simulink model "FOC_HSMO_G474"  (R2020b)
settings: Solver=FixedStepDiscrete  StartTime=0.0  StopTime=10  FixedStep=TsBSP  RelTol=1e-3
PreLoadFcn:
  | a=1;
values from neighbouring files (symbols this model uses):
  BandwidthCurrentPI = 1256.6370614359173    [G474_FOC_HSMO.sldd]
  GainK = 2.0    [G474_FOC_HSMO.sldd]
  GainM = 0.15    [G474_FOC_HSMO.sldd]
  Ld = 0.000195185    [G474_FOC_HSMO.sldd]    (also in Hall_HSMO_FOC_Data.sldd = 0.0004
  Ld_MODEL = 0.000195185    [G474_FOC_HSMO.sldd]
  Lq = 0.000195185    [G474_FOC_HSMO.sldd]    (also in Hall_HSMO_FOC_Data.sldd = 0.00045
  Lq_MODEL = 0.000195185    [G474_FOC_HSMO.sldd]
  MaxVoltage = 10.0    [G474_FOC_HSMO.sldd]
  PolePairs = 5.0    [G474_FOC_HSMO.sldd]
  PolePairs_MODEL = 5.0    [G474_FOC_HSMO.sldd]
  PWMHalfPeriod = 4199.0    [G474_FOC_HSMO.sldd]
  Rs = 0.1764    [G474_FOC_HSMO.sldd]
  TsBSP = 5.0E-6    [G474_FOC_HSMO.sldd]
  TsFOC = 0.0001    [G474_FOC_HSMO.sldd]
  TsFOC_MODEL = 0.0001    [G474_FOC_HSMO.sldd]
undefined symbols (not defined in the file or in its folder): DiscIntNeverNeededParam, sigbuilder_block
libraries: pid_lib x3, mcbplantlib x1, autolibpmsminterior x1
(part 1 of 2)
PreSaveFcn:
  | cd(fileparts(which(bdroot)));
settings Model: DataDictionary=G474_FOC_HSMO.sldd  PauseTimes=1  PacingRate=1.100000  Creator=beau_  LastModifiedBy=Administrator
settings DataIOCC: SaveOutput=off  DSMLogging=off  SaveTime=off  ReturnWorkspaceOutputs=off
settings OptimizationCC: DefaultParameterBehavior=Inlined  EnhancedBackFolding=on  PassReuseOutputArgsAs=Individual arguments  ZeroExternalMemoryAtStartup=off  OptimizeBlockOrder=speed  DifferentSizesBufferReuse=on  OptimizationCustomize=off  EfficientTunableParamExpr=on
settings DebuggingCC: SignalRangeChecking=warning  ParameterPrecisionLossMsg=none  ParameterTunabilityLossMsg=error
settings HardwareCC: ProdBitPerPointer=32  ProdBitPerSizeT=32  ProdBitPerPtrDiffT=32  ProdLargestAtomicInteger=Long  ProdLargestAtomicFloat=Double  ProdWordSize=32  ProdHWDeviceType=ARM Compatible->ARM Cortex-M
settings SFSimCC: SimParseCustomCode=off  MATLABDynamicMemAlloc=off
settings RTWCC: Description=Embedded Coder  SystemTargetFile=ert.tlc  GenCodeOnly=on  TemplateMakefile=ert_default_tmf  RTWUseSimCustomCode=on
settings CodeAppCC: ForceParamTrailComments=on  GenerateComments=off  IgnoreCustomStorageClasses=off  OperatorAnnotations=on  SimulinkDataObjDesc=on  SFDataObjDesc=on  InsertBlockDesc=on
settings ERTTargetCC: TargetLangStandard=C99 (ISO)  CodeReplacementLibrary=ARM Cortex-M  GenerateSampleERTMain=on  SupportAbsoluteTime=off  SupportNonFinite=off  SupportComplex=off  InlinedParameterPlacement=NonHierarchical  ERTCustomFileTemplate=example_file_process.tlc  IndentSize=4

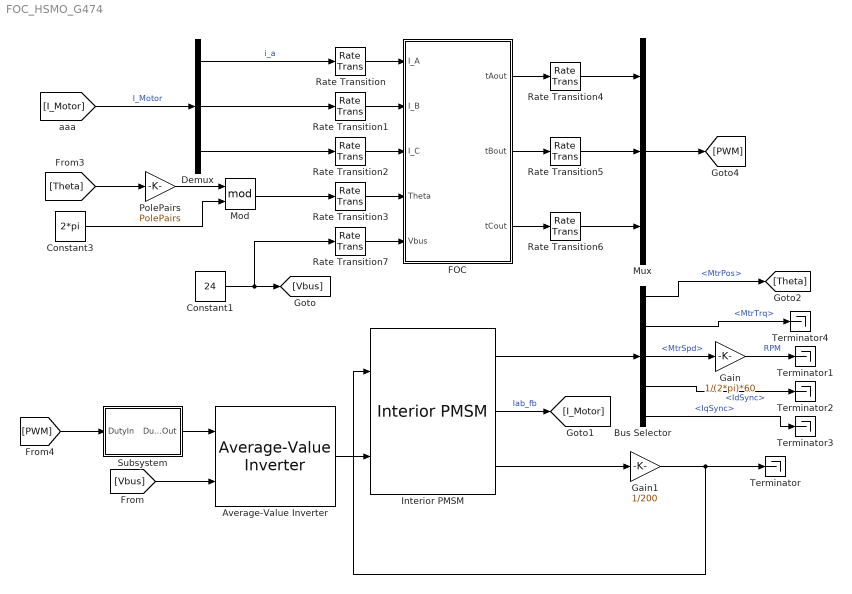
== system FOC_HSMO_G474 ==
  Average-Value Inverter : mcbplantlib/Average-Value Inverter
  Bus Selector : BusSelector  OutputSignals=MtrPos,MtrTrq,MtrSpd,IdSync,IqSync
  Constant1 : Constant  Value=24  SampleTime=TsBSP
  Constant3 : Constant  Value=2*pi  SampleTime=TsBSP
  Demux : Demux  Outputs=3
  FOC : Subsystem  SystemSampleTime=TsFOC
  Gain : Gain  Gain=1/(2*pi)*60
  Gain1 : Gain  Gain=1/200
  Interior PMSM : autolibpmsminterior/Interior PMSM  port_config=Torque  sim_type=Discrete  Ts=TsBSP  P=PolePairs_MODEL  Rs=Rs_MODEL  Ldq=[Ld_MODEL Lq_MODEL]  KConstText=Permanent flux linkage constant (lambda_pm):  lambda_pm=Flux_MODEL  Ke=159.9771  mechanical=[2.8e-4,1e-5,0.01]  idq0=[0 0]  theta_init=0  omega_init=5  KConst=Flux_MODEL  lambda_pm_calc=Flux_MODEL  Kt=0.07  RefBlkName='autolibpmsminterior/Interior PMSM'  aMode=5
      settings: SourceProductBaseCode=PW,MT,UV,VE,VP
  Mod : Math  Operator=mod  SaturateOnIntegerOverflow=on
  Mux : Mux  Inputs=3
  PolePairs : Gain  Gain=PolePairs
  Rate Transition{,1..3,7} (5 alike) : RateTransition
  Rate Transition4 : RateTransition  OutPortSampleTime=TsBSP
  Rate Transition5 : RateTransition  OutPortSampleTime=TsBSP
  Rate Transition6 : RateTransition  OutPortSampleTime=TsBSP
  Subsystem : Subsystem
  Terminator{,1..4} (5 alike) : Terminator
  wires:
  Average-Value Inverter/1 -> Interior PMSM/2
  Rate Transition4/1 -> Mux/1
  Interior PMSM/2 -> [I_Motor]  "Iab_fb"
  Rate Transition7/1 -> FOC/5(Vbus)
  Interior PMSM/3 -> Gain1/1
  Bus Selector/5 -> Terminator3/1  "<IqSync>"
  Bus Selector/4 -> Terminator2/1  "<IdSync>"
  [Vbus] -> Average-Value Inverter/2
  Mux/1 -> [PWM]
  Rate Transition2/1 -> FOC/3(I_C)
  Mod/1 -> Rate Transition3/1
  PolePairs/1 -> Mod/1
  Subsystem/1(DutyOut) -> Average-Value Inverter/1
  Constant1/1 -> Rate Transition7/1, [Vbus]
  Rate Transition3/1 -> FOC/4(Theta)
  Demux/3 -> Rate Transition2/1
  Rate Transition/1 -> FOC/1(I_A)
  Demux/1 -> Rate Transition/1  "i_a"
  Gain1/1 -> Interior PMSM/1, Terminator/1
  Rate Transition5/1 -> Mux/2
  Interior PMSM/1 -> Bus Selector/1
  Rate Transition6/1 -> Mux/3
  Bus Selector/1 -> [Theta]  "<MtrPos>"
  FOC/2(tBout) -> Rate Transition5/1
  [Theta] -> PolePairs/1
  FOC/3(tCout) -> Rate Transition6/1
  FOC/1(tAout) -> Rate Transition4/1
  Demux/2 -> Rate Transition1/1
  Bus Selector/3 -> Gain/1  "<MtrSpd>"
  Constant3/1 -> Mod/2
  Rate Transition1/1 -> FOC/2(I_B)
  [PWM] -> Subsystem/1(DutyIn)
  [I_Motor] -> Demux/1  "I_Motor"
  Gain/1 -> Terminator1/1  "RPM"
  Bus Selector/2 -> Terminator4/1  "<MtrTrq>"

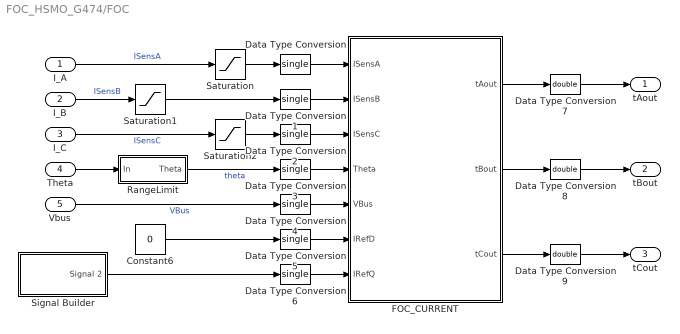
== system FOC_HSMO_G474/FOC ==
  I_A : Inport  OutMin=-100  OutMax=100
  I_B : Inport  Port=2
  I_C : Inport  Port=3
  Theta : Inport  Port=4
  Vbus : Inport  Port=5
  Constant6 : Constant  Value=0  SampleTime=-1
  Data Type Conversion{,1..6} (7 alike) : DataTypeConversion  OutDataTypeStr=single
  Data Type Conversion7 : DataTypeConversion  OutDataTypeStr=double
  Data Type Conversion8 : DataTypeConversion  OutDataTypeStr=double
  Data Type Conversion9 : DataTypeConversion  OutDataTypeStr=double
  FOC_CURRENT : Subsystem  TreatAsAtomicUnit=on  SystemSampleTime=TsFOC_MODEL
  RangeLimit : Subsystem
  Saturation : Saturate  UpperLimit=100  LowerLimit=-100
  Saturation1 : Saturate  UpperLimit=100  LowerLimit=-100
  Saturation2 : Saturate  UpperLimit=100  LowerLimit=-100
  Signal Builder : Subsystem  Tag=STV Subsys  LoadFcn=sigbuilder_block('load');  StartFcn=sigbuilder_block('start');  StopFcn=sigbuilder_block('stop');  ClipboardFcn=sigbuilder_block('clipboard');  mask(Sigbuilder block){tuvar=[0:10]}
      mask help: Simulink:masks:SigbuilderBlock_MD
      mask init:
      | if ~strcmp(get_param(bdroot(gcbh),'SimulationStatus'),'stopped') tuvar = sigbuilder_block('maskInit'); end
      settings: CopyFcn=sigbuilder_block('copy');  DeleteFcn=sigbuilder_block('delete');  ModelCloseFcn=sigbuilder_block('modelClose');  PreSaveFcn=sigbuilder_block('preSave');  PauseFcn=sigbuilder_block('pause');  ContinueFcn=sigbuilder_block('continue');  NameChangeFcn=sigbuilder_block('namechange');  OpenFcn=sigbuilder_block('open',[163.5 909 1141.5 540 ]);  CloseFcn=sigbuilder_block('close');
      mask Display: plot(0, 0, 100, 100,[2, 2, 32, 32, 2], [68, 8, 8, 68, 68],[32, 2], [38, 38], [32, 19, 2],[53, 60, 44], [32, 17, 17, 2],[16, 16, 31, 31]);txt = getActiveGroup(gcbh);text(2, 100, txt,'verticalAlignment', 'top');
  tAout : Outport
  tBout : Outport  Port=2
  tCout : Outport  Port=3
  wires:
  I_A/1 -> Saturation/1  "ISensA"
  I_C/1 -> Saturation2/1  "ISensC"
  Vbus/1 -> Data Type Conversion4/1  "VBus"
  I_B/1 -> Saturation1/1  "ISensB"
  Constant6/1 -> Data Type Conversion5/1
  Theta/1 -> RangeLimit/1(In)
  FOC_CURRENT/3(tCout) -> Data Type Conversion9/1
  FOC_CURRENT/1(tAout) -> Data Type Conversion7/1
  FOC_CURRENT/2(tBout) -> Data Type Conversion8/1
  Saturation/1 -> Data Type Conversion/1
  Saturation1/1 -> Data Type Conversion1/1
  Saturation2/1 -> Data Type Conversion2/1
  RangeLimit/1(Theta) -> Data Type Conversion3/1  "theta"
  Signal Builder/1(Signal 2) -> Data Type Conversion6/1
  Data Type Conversion/1 -> FOC_CURRENT/1(ISensA)
  Data Type Conversion1/1 -> FOC_CURRENT/2(ISensB)
  Data Type Conversion2/1 -> FOC_CURRENT/3(ISensC)
  Data Type Conversion3/1 -> FOC_CURRENT/4(Theta)
  Data Type Conversion4/1 -> FOC_CURRENT/5(VBus)
  Data Type Conversion5/1 -> FOC_CURRENT/6(IRefD)
  Data Type Conversion6/1 -> FOC_CURRENT/7(IRefQ)
  Data Type Conversion7/1 -> tAout/1
  Data Type Conversion8/1 -> tBout/1
  Data Type Conversion9/1 -> tCout/1

== system FOC_HSMO_G474/Subsystem ==
  DutyIn : Inport
  Constant : Constant  Value=0.5  SampleTime=TsBSP
  Gain : Gain  Gain=1/PWMHalfPeriod  ParamDataTypeStr=single
  Gain1 : Gain  Gain=-1
  Sum : Sum  Inputs=|+-
  Sum1 : Sum  Inputs=|++
  DutyOut : Outport
  wires:
  Sum/1 -> Gain1/1
  Constant/1 -> Sum1/2, Sum/2
  DutyIn/1 -> Gain/1
  Gain1/1 -> Sum1/1
  Sum1/1 -> DutyOut/1
  Gain/1 -> Sum/1

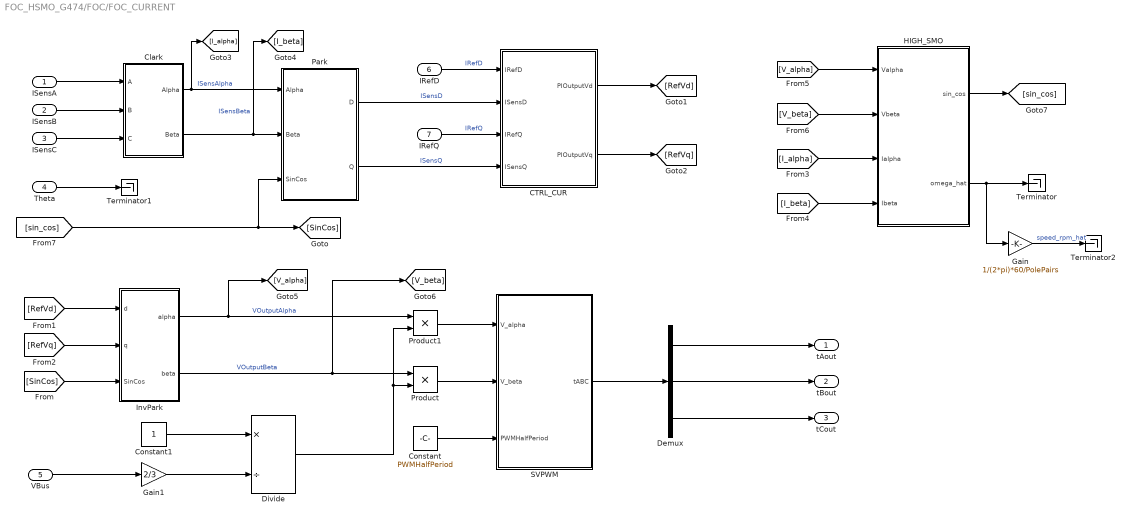
== system FOC_HSMO_G474/FOC/FOC_CURRENT ==
  ISensA : Inport  OutMin=-100  OutMax=100
  ISensB : Inport  Port=2  OutMin=-100  OutMax=100
  ISensC : Inport  Port=3  OutMin=-100  OutMax=100
  Theta : Inport  Port=4  OutMin=-2*pi  OutMax=2*pi
  VBus : Inport  Port=5  OutMin=0  OutMax=500
  IRefD : Inport  Port=6  OutMin=-50  OutMax=50
  IRefQ : Inport  Port=7  OutMin=-50  OutMax=50
  CTRL_CUR : Subsystem  TreatAsAtomicUnit=on
  Clark : Subsystem  TreatAsAtomicUnit=on
      settings: RTWSystemCode=Inline  RTWFcnNameOpts=Use subsystem name
      mask Display:
      | port_label('input',1,'a','texmode','on');
      | port_label('input',2,'b','texmode','on');
      | port_label('input',3,'c','texmode','on');
      | 
      | port_label('output',1,'\alpha','texmode','on');
      | port_label('output',2,'\beta','texmode','on');
      | 
      | fprintf('Clark');
  Constant : Constant  Value=PWMHalfPeriod  OutDataTypeStr=single  SampleTime=-1
  Constant1 : Constant  OutDataTypeStr=single  SampleTime=-1
  Demux : Demux  Outputs=3
  Divide : Product  Inputs=*/
  Gain : Gain  Gain=1/(2*pi)*60/PolePairs
  Gain1 : Gain  Gain=2/3
  HIGH_SMO : Subsystem
      mask Display:
      | port_label('input',1,'U_\alpha','texmode','on');
      | port_label('input',2,'U_\beta','texmode','on');
      | port_label('input',3,'I_\alpha','texmode','on');
      | port_label('input',4,'I_\beta','texmode','on');
      | 
      | port_label('output',1,'sin(\theta_e)cos(\theta_e)','texmode','on');
      | port_label('output',2,'\omega_e','texmode','on');
      | 
      | fprintf('HSMO');
  InvPark : Subsystem  TreatAsAtomicUnit=on
      settings: RTWFcnNameOpts=Use subsystem name
      mask Display:
      | port_label('input',1,'d','texmode','on');
      | port_label('input',2,'q','texmode','on');
      | port_label('input',3,'\theta','texmode','on');
      | 
      | port_label('output',1,'\alpha','texmode','on');
      | port_label('output',2,'\beta','texmode','on');
      | 
      | fprintf('Inverse\nPark')
  Park : Subsystem  TreatAsAtomicUnit=on
      settings: RTWFcnNameOpts=Use subsystem name
      mask Display:
      | port_label('input',1,'\alpha','texmode','on');
      | port_label('input',2, '\beta','texmode','on');
      | port_label('input',3, '\theta','texmode','on');
      | 
      | port_label('output',1,'d','texmode','on');
      | port_label('output',2,'q','texmode','on');
      | fprintf('Park');
  Product : Product
  Product1 : Product
  SVPWM : Subsystem  TreatAsAtomicUnit=on
  Terminator : Terminator
  Terminator1 : Terminator
  Terminator2 : Terminator
  tAout : Outport
  tBout : Outport  Port=2
  tCout : Outport  Port=3
  wires:
  Constant1/1 -> Divide/1
  CTRL_CUR/2(PIOutputVq) -> [RefVq]
  [RefVq] -> InvPark/2(q)
  InvPark/1(alpha) -> Product1/1, [V_alpha]  "VOutputAlpha"
  ISensB/1 -> Clark/2(B)
  IRefQ/1 -> CTRL_CUR/3(IRefQ)  "IRefQ"
  Divide/1 -> Product1/2, Product/2
  Product/1 -> SVPWM/2(V_beta)
  Park/2(Q) -> CTRL_CUR/4(ISensQ)  "ISensQ"
  Gain1/1 -> Divide/2
  [SinCos] -> InvPark/3(SinCos)
  IRefD/1 -> CTRL_CUR/1(IRefD)  "IRefD"
  InvPark/2(beta) -> Product/1, [V_beta]  "VOutputBeta"
  [RefVd] -> InvPark/1(d)
  Constant/1 -> SVPWM/3(PWMHalfPeriod)
  Park/1(D) -> CTRL_CUR/2(ISensD)  "ISensD"
  VBus/1 -> Gain1/1
  CTRL_CUR/1(PIOutputVd) -> [RefVd]
  [sin_cos] -> Park/3(SinCos), [SinCos]
  ISensC/1 -> Clark/3(C)
  ISensA/1 -> Clark/1(A)
  Product1/1 -> SVPWM/1(V_alpha)
  SVPWM/1(tABC) -> Demux/1
  Demux/1 -> tAout/1
  Demux/2 -> tBout/1
  Demux/3 -> tCout/1
  Clark/1(Alpha) -> Park/1(Alpha), [I_alpha]  "ISensAlpha"
  Clark/2(Beta) -> [I_beta], Park/2(Beta)  "ISensBeta"
  [I_alpha] -> HIGH_SMO/3(Ialpha)
  [I_beta] -> HIGH_SMO/4(Ibeta)
  [V_alpha] -> HIGH_SMO/1(Valpha)
  [V_beta] -> HIGH_SMO/2(Vbeta)
  HIGH_SMO/1(sin_cos) -> [sin_cos]
  HIGH_SMO/2(omega_hat) -> Gain/1, Terminator/1
  Gain/1 -> Terminator2/1  "speed_rpm_hat"
  Theta/1 -> Terminator1/1

== system FOC_HSMO_G474/FOC/RangeLimit ==
  In : Inport
  Constant : Constant  Value=2*pi  SampleTime=-1
  Constant1 : Constant  Value=0  SampleTime=-1
  If : If  NumInputs=2  IfExpression=u1  ElseIfExpressions=u2
  If Action Subsystem : Subsystem  TreatAsAtomicUnit=on
  If Action Subsystem1 : Subsystem  TreatAsAtomicUnit=on
  If Action Subsystem2 : Subsystem  TreatAsAtomicUnit=on
  Merge : Merge  Inputs=3
  Relational Operator : RelationalOperator  Operator=>  OutDataTypeStr=boolean  RndMeth=Simplest
  Relational Operator1 : RelationalOperator  Operator=<  OutDataTypeStr=boolean  RndMeth=Simplest
  Theta : Outport
  wires:
  Relational Operator/1 -> If/1
  Constant/1 -> Relational Operator/2
  Constant1/1 -> Relational Operator1/2
  In/1 -> Relational Operator1/1, If Action Subsystem2/1(In1), If Action Subsystem1/1(In1), If Action Subsystem/1(In1), Relational Operator/1
  Relational Operator1/1 -> If/2
  Merge/1 -> Theta/1
  If/3 -> If Action Subsystem2/Action
  If/2 -> If Action Subsystem/Action
  If/1 -> If Action Subsystem1/Action
  If Action Subsystem2/1(Out1) -> Merge/1
  If Action Subsystem/1(Out1) -> Merge/2
  If Action Subsystem1/1(Out1) -> Merge/3

== system FOC_HSMO_G474/FOC/Signal Builder ==
  Demux : Demux  Tag=STV Demux  Outputs=1
      settings: DisplayOption=none
  FromWs : FromWorkspace  Tag=STV FromWs  VariableName=tuvar
      SigBuilderData=|
      | common.afterFinalStr = 'Extrapolate'
      | common.sampleTime = 0
      | dataSet.timeRange = [0 10]
      | dataSet.name = 'Group 1'
      | sbobj.Groups.Name = 'Group 1'
      | sbobj.Groups.Signals.Name = 'Signal 2'
      | sbobj.Groups.Signals.XData = [0 0.99 0.99 1.98 1.98 3 3 4 4 5.01 5.01 6 6 7 7.99 7.99 9 9 10]
      | sbobj.Groups.Signals.YData = [2.85 2.85 8.85 8.85 1.55 1.55 2.7 2.7 9.45 5.25 5.3 5.3 0.8 0.8 0.8 9.95 9.95 10 10]
  Signal 2 : Outport  Tag=STV Outport
  wires:
  FromWs/1 -> Demux/1
  Demux/1 -> Signal 2/1

== system FOC_HSMO_G474/FOC/FOC_CURRENT/CTRL_CUR ==
  IRefD : Inport
  ISensD : Inport  Port=2
  IRefQ : Inport  Port=3
  ISensQ : Inport  Port=4
  Constant1 : Constant  Value=Rs*BandwidthCurrentPI  OutDataTypeStr=single  SampleTime=-1
  Constant2 : Constant  Value=Lq*BandwidthCurrentPI  OutDataTypeStr=single  SampleTime=-1
  Constant3 : Constant  Value=Rs*BandwidthCurrentPI  OutDataTypeStr=single  SampleTime=-1
  Constant4 : Constant  Value=Ld*BandwidthCurrentPI  OutDataTypeStr=single  SampleTime=-1
  Discrete PID Controller : pid_lib/PID Controller  Controller=PI  Form=Parallel  TimeDomain=Discrete-time  UseExternalTs=off  SampleTime=-1  IntegratorMethod=Forward Euler  FilterMethod=Forward Euler  ControllerParametersSource=external  P=1  I=1  D=0  UseFilter=off  N=100  TunerSelectOption=Transfer Function Based (PID Tuner App)  ZeroCross=off  InitialConditionSource=internal  InitialConditionForIntegrator=0  InitialConditionForFilter=0  DifferentiatorICPrevScaledInput=0  ExternalReset=none  TrackingMode=off  Kt=1  LimitOutput=on  SatLimitsSource=internal  UpperSaturationLimit=MaxVoltage  LowerSaturationLimit=-MaxVoltage  LinearizeAsGain=off  AntiWindupMode=clamping  Kb=1  POutMin=[]  POutMax=[]  IOutMin=[]  IOutMax=[]  DOutMin=[]  DOutMax=[]  NOutMin=[]  NOutMax=[]  SumOutMin=[]  SumOutMax=[]  SaturationOutDataTypeStr=Inherit: Inherit via back propagation  SaturationOutMin=[]  SaturationOutMax=[]  PParamMin=[]  PParamMax=[]  IParamMin=[]  IParamMax=[]  DParamMin=[]  DParamMax=[]  NParamMin=[]  NParamMax=[]  KbParamMin=[]  KbParamMax=[]  KtParamMin=[]  KtParamMax=[]  KbOutMin=[]  KbOutMax=[]  KtOutMin=[]  KtOutMax=[]  IntegratorOutMin=[]  IntegratorOutMax=[]  FilterOutMin=[]  FilterOutMax=[]  SumI1OutMin=[]  SumI1OutMax=[]  SumI2OutMin=[]  SumI2OutMax=[]  SumI3OutMin=[]  SumI3OutMax=[]  SumI4OutMin=[]  SumI4OutMax=[]  SumDOutMin=[]  SumDOutMax=[]  DifferentiatorOutMin=[]  DifferentiatorOutMax=[]  FilterDiffOutCoefMin=[]  FilterDiffOutCoefMax=[]  ReciprocalOutMin=[]  ReciprocalOutMax=[]  SumDenOutMin=[]  SumDenOutMax=[]  SumNumOutMin=[]  SumNumOutMax=[]  DivideOutMin=[]  DivideOutMax=[]  UdiffTsProdOutMin=[]  UdiffTsProdOutMax=[]  NTsProdOutMin=[]  NTsProdOutMax=[]  UintegralTsProdOutMin=[]  UintegralTsProdOutMax=[]  UngainTsProdOutMin=[]  UngainTsProdOutMax=[]  IntegratorContinuousStateAttributes=''  IntegratorStateMustResolveToSignalObject=off  IntegratorRTWStateStorageClass=Auto  FilterContinuousStateAttributes=''  FilterStateMustResolveToSignalObject=off  FilterRTWStateStorageClass=Auto  ParallelPVariant=ExternalParameters  IdealPVariant=Disabled  IVariant=ExternalParameters  DVariant=Disabled  IntegratorVariant=Discrete  SatVariant=Enabled  AWVariant=DiscClampingParallel  PCopyVariant=Disabled  TRVariant=Disabled  FdbkBlocksVariant=Forward  IdealPFdbkVariant=Disabled  SatFdbkVariant=Disabled  DerivativeFilterVariant=Disabled  NVariant=Disabled  NCopyVariant=Disabled_SignalSpec  FilterICVariant=Disabled  IntegratorICVariant=InternalICs  ExternalResetVariant=Disabled  TRSumVariant=Passthrough  SumFdbkVariant=Disabled  SumVariant=Sum_PI  TsampFilterVariant=InternalTs  TsampNgainVariant=Passthrough  TsampIntegralVariant=Passthrough  ExternalSaturationOutDataTypeStr=Inherit: Same as second input
  Discrete PID Controller1 : pid_lib/PID Controller  Controller=PI  Form=Parallel  TimeDomain=Discrete-time  UseExternalTs=off  SampleTime=-1  IntegratorMethod=Forward Euler  FilterMethod=Forward Euler  ControllerParametersSource=external  P=1  I=1  D=0  UseFilter=off  N=100  TunerSelectOption=Transfer Function Based (PID Tuner App)  ZeroCross=off  InitialConditionSource=internal  InitialConditionForIntegrator=0  InitialConditionForFilter=0  DifferentiatorICPrevScaledInput=0  ExternalReset=none  TrackingMode=off  Kt=1  LimitOutput=on  SatLimitsSource=internal  UpperSaturationLimit=MaxVoltage  LowerSaturationLimit=-MaxVoltage  LinearizeAsGain=off  AntiWindupMode=clamping  Kb=1  POutMin=[]  POutMax=[]  IOutMin=[]  IOutMax=[]  DOutMin=[]  DOutMax=[]  NOutMin=[]  NOutMax=[]  SumOutMin=[]  SumOutMax=[]  SaturationOutDataTypeStr=Inherit: Inherit via back propagation  SaturationOutMin=[]  SaturationOutMax=[]  PParamMin=[]  PParamMax=[]  IParamMin=[]  IParamMax=[]  DParamMin=[]  DParamMax=[]  NParamMin=[]  NParamMax=[]  KbParamMin=[]  KbParamMax=[]  KtParamMin=[]  KtParamMax=[]  KbOutMin=[]  KbOutMax=[]  KtOutMin=[]  KtOutMax=[]  IntegratorOutMin=[]  IntegratorOutMax=[]  FilterOutMin=[]  FilterOutMax=[]  SumI1OutMin=[]  SumI1OutMax=[]  SumI2OutMin=[]  SumI2OutMax=[]  SumI3OutMin=[]  SumI3OutMax=[]  SumI4OutMin=[]  SumI4OutMax=[]  SumDOutMin=[]  SumDOutMax=[]  DifferentiatorOutMin=[]  DifferentiatorOutMax=[]  FilterDiffOutCoefMin=[]  FilterDiffOutCoefMax=[]  ReciprocalOutMin=[]  ReciprocalOutMax=[]  SumDenOutMin=[]  SumDenOutMax=[]  SumNumOutMin=[]  SumNumOutMax=[]  DivideOutMin=[]  DivideOutMax=[]  UdiffTsProdOutMin=[]  UdiffTsProdOutMax=[]  NTsProdOutMin=[]  NTsProdOutMax=[]  UintegralTsProdOutMin=[]  UintegralTsProdOutMax=[]  UngainTsProdOutMin=[]  UngainTsProdOutMax=[]  IntegratorContinuousStateAttributes=''  IntegratorStateMustResolveToSignalObject=off  IntegratorRTWStateStorageClass=Auto  FilterContinuousStateAttributes=''  FilterStateMustResolveToSignalObject=off  FilterRTWStateStorageClass=Auto  ParallelPVariant=ExternalParameters  IdealPVariant=Disabled  IVariant=ExternalParameters  DVariant=Disabled  IntegratorVariant=Discrete  SatVariant=Enabled  AWVariant=DiscClampingParallel  PCopyVariant=Disabled  TRVariant=Disabled  FdbkBlocksVariant=Forward  IdealPFdbkVariant=Disabled  SatFdbkVariant=Disabled  DerivativeFilterVariant=Disabled  NVariant=Disabled  NCopyVariant=Disabled_SignalSpec  FilterICVariant=Disabled  IntegratorICVariant=InternalICs  ExternalResetVariant=Disabled  TRSumVariant=Passthrough  SumFdbkVariant=Disabled  SumVariant=Sum_PI  TsampFilterVariant=InternalTs  TsampNgainVariant=Passthrough  TsampIntegralVariant=Passthrough  ExternalSaturationOutDataTypeStr=Inherit: Same as second input
  Sum : Sum  Inputs=|+-
  Sum1 : Sum  Inputs=|+-
  PIOutputVd : Outport
  PIOutputVq : Outport  Port=2
  wires:
  IRefD/1 -> Sum/1
  Sum/1 -> Discrete PID Controller/1
  Discrete PID Controller/1 -> PIOutputVd/1  "PIOutputVd"
  ISensD/1 -> Sum/2
  Constant4/1 -> Discrete PID Controller/2
  Constant3/1 -> Discrete PID Controller/3
  IRefQ/1 -> Sum1/1
  Constant2/1 -> Discrete PID Controller1/2
  Sum1/1 -> Discrete PID Controller1/1
  ISensQ/1 -> Sum1/2
  Constant1/1 -> Discrete PID Controller1/3
  Discrete PID Controller1/1 -> PIOutputVq/1  "PIOutputVq"

== system FOC_HSMO_G474/FOC/FOC_CURRENT/Clark ==
  A : Inport
  B : Inport  Port=2
  C : Inport  Port=3
  Gain : Gain  Gain=single(2/3)
  Gain1 : Gain  Gain=0.5
  Gain2 : Gain  Gain=single(sqrt(3)/3)
  Sum : Sum  Inputs=|++
  Sum1 : Sum  Inputs=|+-
  Sum2 : Sum  Inputs=+-|
  Alpha : Outport
  Beta : Outport  Port=2
  wires:
  Sum/1 -> Gain1/1
  Gain2/1 -> Beta/1
  B/1 -> Sum2/1, Sum/1
  Gain1/1 -> Sum1/2
  Gain/1 -> Alpha/1
  Sum2/1 -> Gain2/1
  C/1 -> Sum2/2, Sum/2
  A/1 -> Sum1/1
  Sum1/1 -> Gain/1

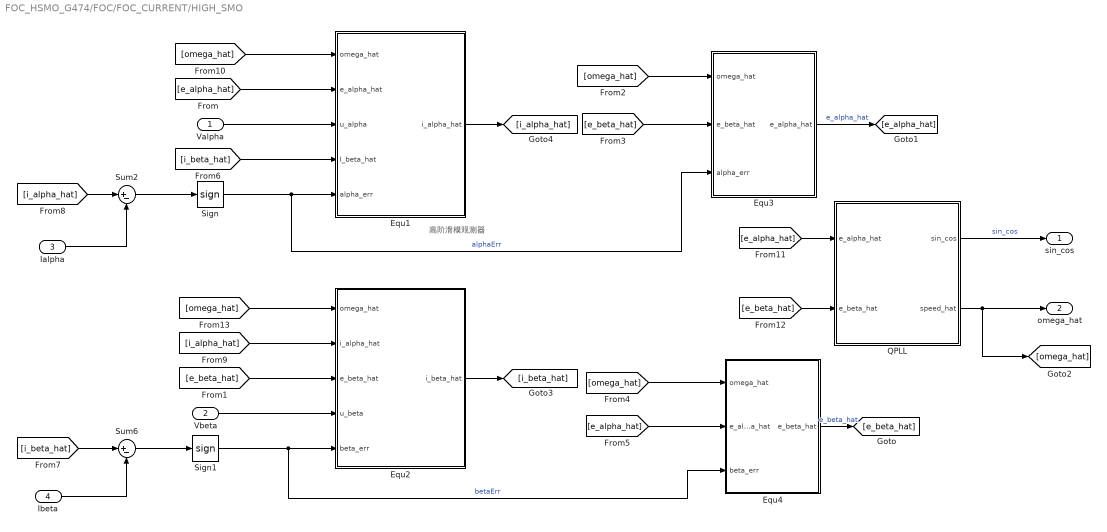
== system FOC_HSMO_G474/FOC/FOC_CURRENT/HIGH_SMO ==
  note: 高阶滑模观测器
  Valpha : Inport
  Vbeta : Inport  Port=2
  Ialpha : Inport  Port=3
  Ibeta : Inport  Port=4
  Equ1 : Subsystem
  Equ2 : Subsystem
  Equ3 : Subsystem
  Equ4 : Subsystem
  QPLL : Subsystem
  Sign : Signum
  Sign1 : Signum
  Sum2 : Sum  Inputs=|+-
  Sum6 : Sum  Inputs=|+-
  sin_cos : Outport
  omega_hat : Outport  Port=2
  wires:
  Sum6/1 -> Sign1/1
  Sum2/1 -> Sign/1
  Sign/1 -> Equ3/3(alpha_err), Equ1/5(alpha_err)  "alphaErr"
  Ialpha/1 -> Sum2/2
  Sign1/1 -> Equ4/3(beta_err), Equ2/5(beta_err)  "betaErr"
  Ibeta/1 -> Sum6/2
  Equ1/1(i_alpha_hat) -> [i_alpha_hat]
  [e_alpha_hat] -> Equ1/2(e_alpha_hat)
  Valpha/1 -> Equ1/3(u_alpha)
  [e_beta_hat] -> Equ2/3(e_beta_hat)
  Vbeta/1 -> Equ2/4(u_beta)
  Equ2/1(i_beta_hat) -> [i_beta_hat]
  [i_beta_hat] -> Equ1/4(I_beta_hat)
  [i_beta_hat] -> Sum6/1
  [i_alpha_hat] -> Sum2/1
  [i_alpha_hat] -> Equ2/2(i_alpha_hat)
  [omega_hat] -> Equ3/1(omega_hat)
  [e_beta_hat] -> Equ3/2(e_beta_hat)
  [omega_hat] -> Equ4/1(omega_hat)
  [e_alpha_hat] -> Equ4/2(e_alpha_hat)
  [omega_hat] -> Equ1/1(omega_hat)
  Equ4/1(e_beta_hat) -> [e_beta_hat]  "e_beta_hat"
  Equ3/1(e_alpha_hat) -> [e_alpha_hat]  "e_alpha_hat"
  [e_alpha_hat] -> QPLL/1(e_alpha_hat)
  [e_beta_hat] -> QPLL/2(e_beta_hat)
  QPLL/2(speed_hat) -> [omega_hat], omega_hat/1
  QPLL/1(sin_cos) -> sin_cos/1  "sin_cos"
  [omega_hat] -> Equ2/1(omega_hat)

== system FOC_HSMO_G474/FOC/FOC_CURRENT/InvPark ==
  d : Inport
  q : Inport  Port=2
  SinCos : Inport  Port=3
  Demux : Demux  Outputs=2
  Product{,1..3} (4 alike) : Product
  Sum : Sum  Inputs=|+-
  Sum1 : Sum  Inputs=|++
  alpha : Outport
  beta : Outport  Port=2
  wires:
  Sum/1 -> alpha/1
  SinCos/1 -> Demux/1
  d/1 -> Product2/1, Product/1
  Demux/2 -> Product/2, Product3/2
  q/1 -> Product3/1, Product1/1
  Demux/1 -> Product1/2, Product2/2
  Product/1 -> Sum/1
  Product1/1 -> Sum/2
  Product2/1 -> Sum1/1
  Product3/1 -> Sum1/2
  Sum1/1 -> beta/1

== system FOC_HSMO_G474/FOC/FOC_CURRENT/Park ==
  Alpha : Inport
  Beta : Inport  Port=2
  SinCos : Inport  Port=3
  Demux : Demux  Outputs=2
  Product{,1..3} (4 alike) : Product
  Sum : Sum  Inputs=|++
  Sum1 : Sum  Inputs=|-+
  D : Outport
  Q : Outport  Port=2
  wires:
  Beta/1 -> Product3/1, Product1/1
  Alpha/1 -> Product2/1, Product/1
  SinCos/1 -> Demux/1
  Demux/2 -> Product/2, Product3/2
  Demux/1 -> Product1/2, Product2/2
  Product/1 -> Sum/1
  Product1/1 -> Sum/2
  Sum/1 -> D/1
  Product2/1 -> Sum1/1
  Product3/1 -> Sum1/2
  Sum1/1 -> Q/1

== system FOC_HSMO_G474/FOC/FOC_CURRENT/SVPWM ==
  V_alpha : Inport
  V_beta : Inport  Port=2
  PWMHalfPeriod : Inport  Port=3
  CalcPWM : Subsystem
  JudgeSector : Subsystem
  tABC : Outport
  wires:
  V_alpha/1 -> CalcPWM/1(u_alpha_prime), JudgeSector/1(u_alpha_prime)
  V_beta/1 -> CalcPWM/2(u_beta_prime), JudgeSector/2(u_beta_prime)
  JudgeSector/1(sector) -> CalcPWM/3(sector)
  CalcPWM/1(tABC) -> tABC/1
  PWMHalfPeriod/1 -> CalcPWM/4(Tpwm)

== system FOC_HSMO_G474/FOC/RangeLimit/If Action Subsystem ==
  In1 : Inport
  Action Port : ActionPort  ActionPortLabel=elseif(u2)
  Constant : Constant  Value=2*pi  SampleTime=-1
  Sum : Sum  Inputs=|++
  Out1 : Outport
  wires:
  In1/1 -> Sum/1
  Constant/1 -> Sum/2
  Sum/1 -> Out1/1

== system FOC_HSMO_G474/FOC/RangeLimit/If Action Subsystem1 ==
  In1 : Inport
  Action Port : ActionPort  ActionPortLabel=if(u1)
  Constant : Constant  Value=2*pi  SampleTime=-1
  Sum : Sum  Inputs=|+-
  Out1 : Outport
  wires:
  In1/1 -> Sum/1
  Constant/1 -> Sum/2
  Sum/1 -> Out1/1

== system FOC_HSMO_G474/FOC/RangeLimit/If Action Subsystem2 ==
  In1 : Inport
  Action Port : ActionPort  ActionPortLabel=else
  Out1 : Outport
  wires:
  In1/1 -> Out1/1

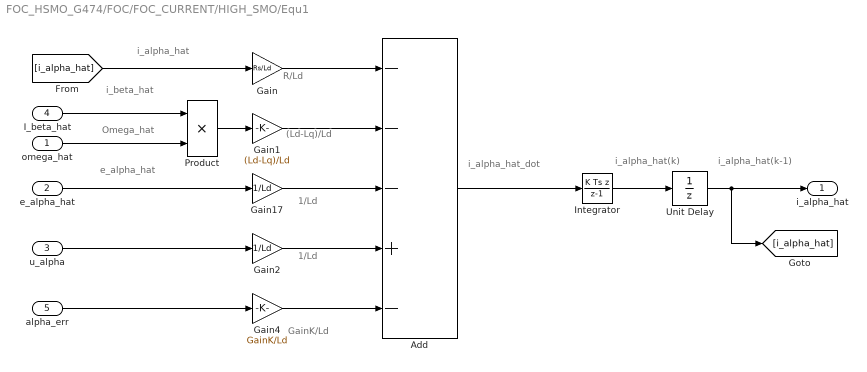
== system FOC_HSMO_G474/FOC/FOC_CURRENT/HIGH_SMO/Equ1 ==
  note: i_alpha_hat(k)
  note: GainK/Ld
  note: i_alpha_hat
  note: R/Ld
  note: (Ld-Lq)/Ld
  note: i_alpha_hat_dot
  note: 1/Ld
  note: e_alpha_hat
  note: 1/Ld
  note: i_beta_hat
  note: Omega_hat
  note: i_alpha_hat(k-1)
  omega_hat : Inport
  e_alpha_hat : Inport  Port=2
  u_alpha : Inport  Port=3
  I_beta_hat : Inport  Port=4
  alpha_err : Inport  Port=5
  Add : Sum  Inputs=---+-
  Gain : Gain  Gain=Rs/Ld
  Gain1 : Gain  Gain=(Ld-Lq)/Ld
  Gain17 : Gain  Gain=1/Ld
  Gain2 : Gain  Gain=1/Ld
  Gain4 : Gain  Gain=GainK/Ld
  Integrator : DiscreteIntegrator  IntegratorMethod=Integration: Backward Euler  SampleTime=-1  ICPrevOutput=DiscIntNeverNeededParam  ICPrevScaledInput=DiscIntNeverNeededParam  mask(DiscretizedDiscreteIntegrator){}
      mask init:
      | %tustin
  Product : Product
  Unit Delay : UnitDelay  SampleTime=-1  HasFrameUpgradeWarning=on
  i_alpha_hat : Outport
  wires:
  Gain1/1 -> Add/2
  Gain4/1 -> Add/5
  Product/1 -> Gain1/1
  Add/1 -> Integrator/1
  I_beta_hat/1 -> Product/1
  Unit Delay/1 -> [i_alpha_hat], i_alpha_hat/1
  Gain/1 -> Add/1
  u_alpha/1 -> Gain2/1
  Gain2/1 -> Add/4
  Integrator/1 -> Unit Delay/1
  omega_hat/1 -> Product/2
  Gain17/1 -> Add/3
  e_alpha_hat/1 -> Gain17/1
  alpha_err/1 -> Gain4/1
  [i_alpha_hat] -> Gain/1

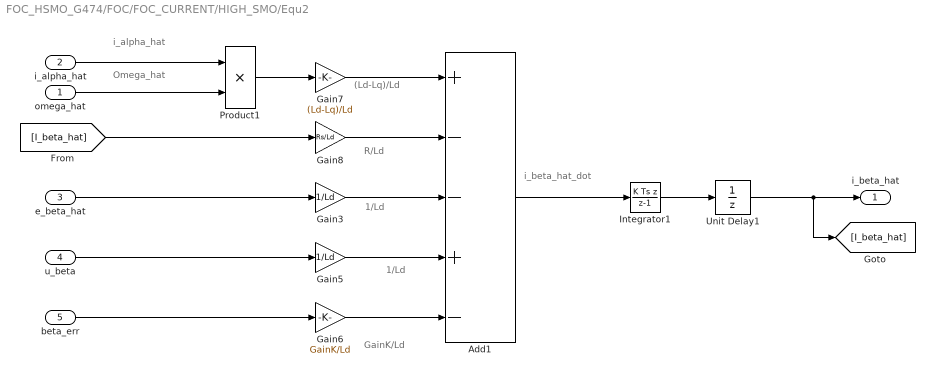
== system FOC_HSMO_G474/FOC/FOC_CURRENT/HIGH_SMO/Equ2 ==
  note: R/Ld
  note: (Ld-Lq)/Ld
  note: 1/Ld
  note: i_alpha_hat
  note: Omega_hat
  note: 1/Ld
  note: GainK/Ld
  note: i_beta_hat_dot
  omega_hat : Inport
  i_alpha_hat : Inport  Port=2
  e_beta_hat : Inport  Port=3
  u_beta : Inport  Port=4
  beta_err : Inport  Port=5
  Add1 : Sum  Inputs=+--+-
  Gain3 : Gain  Gain=1/Ld
  Gain5 : Gain  Gain=1/Ld
  Gain6 : Gain  Gain=GainK/Ld
  Gain7 : Gain  Gain=(Ld-Lq)/Ld
  Gain8 : Gain  Gain=Rs/Ld
  Integrator1 : DiscreteIntegrator  IntegratorMethod=Integration: Backward Euler  SampleTime=-1  ICPrevOutput=DiscIntNeverNeededParam  ICPrevScaledInput=DiscIntNeverNeededParam  mask(DiscretizedDiscreteIntegrator){}
      mask init:
      | %tustin
  Product1 : Product
  Unit Delay1 : UnitDelay  SampleTime=-1  HasFrameUpgradeWarning=on
  i_beta_hat : Outport
  wires:
  Gain8/1 -> Add1/2
  u_beta/1 -> Gain5/1
  Add1/1 -> Integrator1/1
  Gain3/1 -> Add1/3
  i_alpha_hat/1 -> Product1/1
  Gain5/1 -> Add1/4
  Gain6/1 -> Add1/5
  Integrator1/1 -> Unit Delay1/1
  Product1/1 -> Gain7/1
  Gain7/1 -> Add1/1
  beta_err/1 -> Gain6/1
  e_beta_hat/1 -> Gain3/1
  Unit Delay1/1 -> [I_beta_hat], i_beta_hat/1
  omega_hat/1 -> Product1/2
  [I_beta_hat] -> Gain8/1

== system FOC_HSMO_G474/FOC/FOC_CURRENT/HIGH_SMO/Equ3 ==
  note: GainM/Ld
  note: e_alpha_hat_dot
  omega_hat : Inport
  e_beta_hat : Inport  Port=2
  alpha_err : Inport  Port=3
  Add2 : Sum  Inputs=-+
  Gain9 : Gain  Gain=GainM/Ld
  Integrator2 : DiscreteIntegrator  IntegratorMethod=Integration: Backward Euler  SampleTime=-1  ICPrevOutput=DiscIntNeverNeededParam  ICPrevScaledInput=DiscIntNeverNeededParam  mask(DiscretizedDiscreteIntegrator){}
      mask init:
      | %tustin
  Product2 : Product
  Unit Delay2 : UnitDelay  SampleTime=-1  HasFrameUpgradeWarning=on
  e_alpha_hat : Outport
  wires:
  alpha_err/1 -> Gain9/1
  Add2/1 -> Integrator2/1
  Unit Delay2/1 -> e_alpha_hat/1
  omega_hat/1 -> Product2/1
  Product2/1 -> Add2/1
  Integrator2/1 -> Unit Delay2/1
  e_beta_hat/1 -> Product2/2
  Gain9/1 -> Add2/2

== system FOC_HSMO_G474/FOC/FOC_CURRENT/HIGH_SMO/Equ4 ==
  note: GainM/Ld
  note: e_beta_hat_dot
  omega_hat : Inport
  e_alpha_hat : Inport  Port=2
  beta_err : Inport  Port=3
  Add3 : Sum
  Gain10 : Gain  Gain=GainM/Ld
  Integrator3 : DiscreteIntegrator  IntegratorMethod=Integration: Backward Euler  SampleTime=-1  ICPrevOutput=DiscIntNeverNeededParam  ICPrevScaledInput=DiscIntNeverNeededParam  mask(DiscretizedDiscreteIntegrator){}
      mask init:
      | %tustin
  Product3 : Product
  Unit Delay3 : UnitDelay  SampleTime=-1  HasFrameUpgradeWarning=on
  e_beta_hat : Outport
  wires:
  Integrator3/1 -> Unit Delay3/1
  Add3/1 -> Integrator3/1
  Gain10/1 -> Add3/2
  Product3/1 -> Add3/1
  beta_err/1 -> Gain10/1
  Unit Delay3/1 -> e_beta_hat/1
  omega_hat/1 -> Product3/1
  e_alpha_hat/1 -> Product3/2

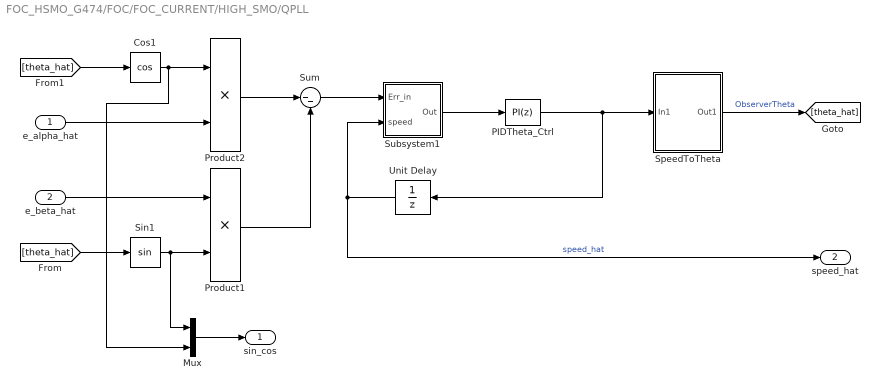
== system FOC_HSMO_G474/FOC/FOC_CURRENT/HIGH_SMO/QPLL ==
  e_alpha_hat : Inport
  e_beta_hat : Inport  Port=2
  Cos1 : Trigonometry  Operator=cos
  Mux : Mux  Inputs=2
  PIDTheta_Ctrl : pid_lib/PID Controller  Controller=PI  Form=Parallel  TimeDomain=Discrete-time  UseExternalTs=off  SampleTime=-1  IntegratorMethod=Forward Euler  FilterMethod=Forward Euler  ControllerParametersSource=internal  P=2*0.707*100  I=100*100  D=0  UseFilter=on  N=100  TunerSelectOption=Transfer Function Based (PID Tuner App)  ZeroCross=off  InitialConditionSource=internal  InitialConditionForIntegrator=1  InitialConditionForFilter=0  DifferentiatorICPrevScaledInput=0  ExternalReset=none  TrackingMode=off  Kt=1  LimitOutput=on  SatLimitsSource=internal  UpperSaturationLimit=2*pi*500  LowerSaturationLimit=-2*pi*500  LinearizeAsGain=off  AntiWindupMode=clamping  Kb=50  POutMin=[]  POutMax=[]  IOutMin=[]  IOutMax=[]  DOutMin=[]  DOutMax=[]  NOutMin=[]  NOutMax=[]  SumOutMin=[]  SumOutMax=[]  SaturationOutDataTypeStr=Inherit: Inherit via back propagation  SaturationOutMin=[]  SaturationOutMax=[]  PParamMin=[]  PParamMax=[]  IParamMin=[]  IParamMax=[]  DParamMin=[]  DParamMax=[]  NParamMin=[]  NParamMax=[]  KbParamMin=[]  KbParamMax=[]  KtParamMin=[]  KtParamMax=[]  KbOutMin=[]  KbOutMax=[]  KtOutMin=[]  KtOutMax=[]  IntegratorOutMin=[]  IntegratorOutMax=[]  FilterOutMin=[]  FilterOutMax=[]  SumI1OutMin=[]  SumI1OutMax=[]  SumI2OutMin=[]  SumI2OutMax=[]  SumI3OutMin=[]  SumI3OutMax=[]  SumI4OutMin=[]  SumI4OutMax=[]  SumDOutMin=[]  SumDOutMax=[]  DifferentiatorOutMin=[]  DifferentiatorOutMax=[]  FilterDiffOutCoefMin=[]  FilterDiffOutCoefMax=[]  ReciprocalOutMin=[]  ReciprocalOutMax=[]  SumDenOutMin=[]  SumDenOutMax=[]  SumNumOutMin=[]  SumNumOutMax=[]  DivideOutMin=[]  DivideOutMax=[]  UdiffTsProdOutMin=[]  UdiffTsProdOutMax=[]  NTsProdOutMin=[]  NTsProdOutMax=[]  UintegralTsProdOutMin=[]  UintegralTsProdOutMax=[]  UngainTsProdOutMin=[]  UngainTsProdOutMax=[]  IntegratorContinuousStateAttributes=''  IntegratorStateMustResolveToSignalObject=off  IntegratorRTWStateStorageClass=Auto  FilterContinuousStateAttributes=''  FilterStateMustResolveToSignalObject=off  FilterRTWStateStorageClass=Auto  ParallelPVariant=InternalParameters  IdealPVariant=Disabled  IVariant=InternalParameters  DVariant=Disabled  IntegratorVariant=Discrete  SatVariant=Enabled  AWVariant=DiscClampingParallel  PCopyVariant=Disabled  TRVariant=Disabled  FdbkBlocksVariant=Forward  IdealPFdbkVariant=Disabled  SatFdbkVariant=Disabled  DerivativeFilterVariant=Disabled  NVariant=Disabled  NCopyVariant=Disabled_SignalSpec  FilterICVariant=Disabled  IntegratorICVariant=InternalICs  ExternalResetVariant=Disabled  TRSumVariant=Passthrough  SumFdbkVariant=Disabled  SumVariant=Sum_PI  TsampFilterVariant=InternalTs  TsampNgainVariant=Passthrough  TsampIntegralVariant=Passthrough  ExternalSaturationOutDataTypeStr=Inherit: Same as second input
  Product1 : Product
  Product2 : Product
  Sin1 : Trigonometry
  SpeedToTheta : Subsystem
  Subsystem1 : Subsystem
  Sum : Sum  Inputs=|--
  Unit Delay : UnitDelay  SampleTime=-1  HasFrameUpgradeWarning=on
  sin_cos : Outport
  speed_hat : Outport  Port=2
  wires:
  Sin1/1 -> Mux/1, Product1/2
  Subsystem1/1(Out) -> PIDTheta_Ctrl/1
  Cos1/1 -> Mux/2, Product2/1
  Sum/1 -> Subsystem1/1(Err_in)
  Product1/1 -> Sum/2
  Product2/1 -> Sum/1
  e_beta_hat/1 -> Product1/1
  e_alpha_hat/1 -> Product2/2
  Unit Delay/1 -> speed_hat/1, Subsystem1/2(speed)  "speed_hat"
  [theta_hat] -> Sin1/1
  [theta_hat] -> Cos1/1
  SpeedToTheta/1(Out1) -> [theta_hat]  "ObserverTheta"
  PIDTheta_Ctrl/1 -> Unit Delay/1, SpeedToTheta/1(In1)
  Mux/1 -> sin_cos/1

== system FOC_HSMO_G474/FOC/FOC_CURRENT/SVPWM/CalcPWM ==
  u_alpha_prime : Inport
  u_beta_prime : Inport  Port=2
  sector : Inport  Port=3
  Tpwm : Inport  Port=4
  Merge : Merge  Inputs=6
  Switch Case : SwitchCase  CaseConditions={1,2,3,4,5,6}  ShowDefaultCase=off
  Switch Case Action Subsystem : Subsystem  TreatAsAtomicUnit=on
  Switch Case Action Subsystem1 : Subsystem  TreatAsAtomicUnit=on
  Switch Case Action Subsystem2 : Subsystem  TreatAsAtomicUnit=on
  Switch Case Action Subsystem3 : Subsystem  TreatAsAtomicUnit=on
  Switch Case Action Subsystem4 : Subsystem  TreatAsAtomicUnit=on
  Switch Case Action Subsystem5 : Subsystem  TreatAsAtomicUnit=on
  tABC : Outport
  wires:
  sector/1 -> Switch Case/1
  Switch Case/1 -> Switch Case Action Subsystem/Action
  u_alpha_prime/1 -> Switch Case Action Subsystem5/1(u_alpha_prime), Switch Case Action Subsystem2/1(u_alpha_prime), Switch Case Action Subsystem1/1(u_alpha_prime), Switch Case Action Subsystem/1(u_alpha_prime), Switch Case Action Subsystem3/1(u_alpha_prime), Switch Case Action Subsystem4/1(u_alpha_prime)
  Tpwm/1 -> Switch Case Action Subsystem5/3(Tpwm), Switch Case Action Subsystem4/3(Tpwm), Switch Case Action Subsystem3/3(Tpwm), Switch Case Action Subsystem2/3(Tpwm), Switch Case Action Subsystem1/3(Tpwm), Switch Case Action Subsystem/3(Tpwm)
  Switch Case/2 -> Switch Case Action Subsystem1/Action
  Switch Case/3 -> Switch Case Action Subsystem2/Action
  Switch Case/4 -> Switch Case Action Subsystem3/Action
  Switch Case/5 -> Switch Case Action Subsystem4/Action
  Switch Case/6 -> Switch Case Action Subsystem5/Action
  u_beta_prime/1 -> Switch Case Action Subsystem5/2(u_beta_prime), Switch Case Action Subsystem4/2(u_beta_prime), Switch Case Action Subsystem3/2(u_beta_prime), Switch Case Action Subsystem/2(u_beta_prime), Switch Case Action Subsystem1/2(u_beta_prime), Switch Case Action Subsystem2/2(u_beta_prime)
  Switch Case Action Subsystem/1(tABC) -> Merge/1
  Switch Case Action Subsystem1/1(tABC) -> Merge/2
  Switch Case Action Subsystem2/1(tABC) -> Merge/3
  Switch Case Action Subsystem3/1(tABC) -> Merge/4
  Switch Case Action Subsystem4/1(tABC) -> Merge/5
  Switch Case Action Subsystem5/1(tABC) -> Merge/6
  Merge/1 -> tABC/1

== system FOC_HSMO_G474/FOC/FOC_CURRENT/SVPWM/JudgeSector ==
  note: $if(u_\beta>0)\\ \quad if(u_\alpha>0)\\ \qquad if(\frac{1}{\sqrt{3}}u_\beta>u_\alpha)\\ \quad \qquad sector=2\\ \qquad else \\ \quad \qquad sector=1\\ \quad else \\ \qquad if(-\frac{1}{\sqrt{3}}u_\beta>u_\alpha)\\ \quad \qquad sector=3\\ \qquad else\\ \quad \qquad secotr = 2\\ else\\ \quad if(u_\alpha>0)\\ \qquad if(\frac{1}{\sqrt{3}}u_\beta>u_\alpha)\\ \quad \qquad sector = 5\\ \qquad else\\ \quad \qquad sector = 6\\ \quad else \\ \qquad if(\frac{1}{\sqrt{3}}u_\beta>u_\alpha)\\ \quad \qquad sector = 4\\ \qquad else\\ \quad \qquad sector = 5$
  u_alpha_prime : Inport
  u_beta_prime : Inport  Port=2
  Constant : Constant  Value=0
  If : If  IfExpression=u1
  If Action Subsystem : Subsystem  TreatAsAtomicUnit=on
  If Action Subsystem1 : Subsystem  TreatAsAtomicUnit=on
  Merge : Merge
  Relational Operator : RelationalOperator  Operator=>  OutDataTypeStr=boolean  RndMeth=Simplest
  sector : Outport
  wires:
  u_beta_prime/1 -> If Action Subsystem1/2(u_beta_prime), If Action Subsystem/2(u_beta_prime), Relational Operator/1
  Constant/1 -> Relational Operator/2
  Relational Operator/1 -> If/1
  If/1 -> If Action Subsystem/Action
  If/2 -> If Action Subsystem1/Action
  u_alpha_prime/1 -> If Action Subsystem1/1(u_alpha_prime), If Action Subsystem/1(u_alpha_prime)
  If Action Subsystem/1(sector) -> Merge/1
  If Action Subsystem1/1(sector) -> Merge/2
  Merge/1 -> sector/1

== system FOC_HSMO_G474/FOC/FOC_CURRENT/HIGH_SMO/QPLL/SpeedToTheta ==
  In1 : Inport
  RangeLimit : Subsystem
  Sum1 : Sum  Inputs=|++
  Ts : Gain  Gain=TsFOC
  Unit Delay : UnitDelay  SampleTime=-1  HasFrameUpgradeWarning=on
  Out1 : Outport
  wires:
  In1/1 -> Ts/1
  Ts/1 -> Sum1/1
  Sum1/1 -> RangeLimit/1(In)
  Unit Delay/1 -> Out1/1, Sum1/2
  RangeLimit/1(Theta) -> Unit Delay/1

== system FOC_HSMO_G474/FOC/FOC_CURRENT/HIGH_SMO/QPLL/Subsystem1 ==
  Err_in : Inport
  speed : Inport  Port=2
  If : If
  If Action Subsystem : Subsystem  TreatAsAtomicUnit=on
  If Action Subsystem1 : Subsystem  TreatAsAtomicUnit=on
  Merge : Merge
  Product : Product
  Out : Outport  VectorParamsAs1DForOutWhenUnconnected=off
  wires:
  speed/1 -> If/1
  Merge/1 -> Product/1
  Err_in/1 -> Product/2
  Product/1 -> Out/1
  If/1 -> If Action Subsystem/Action
  If Action Subsystem/1(Out1) -> Merge/1
  If Action Subsystem1/1(Out1) -> Merge/2
  If/2 -> If Action Subsystem1/Action

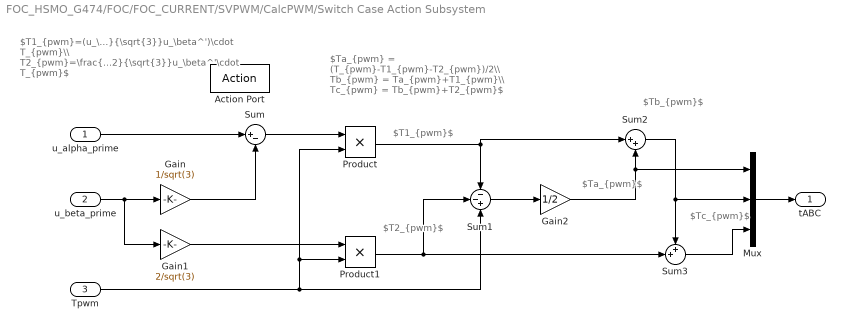
== system FOC_HSMO_G474/FOC/FOC_CURRENT/SVPWM/CalcPWM/Switch Case Action Subsystem ==
  note: $T2_{pwm}$
  note: $T1_{pwm}=(u_\alpha^'-\frac{1}{\sqrt{3}}u_\beta^')\cdot T_{pwm}\\ T2_{pwm}=\frac{2}{\sqrt{3}}u_\beta^'\cdot T_{pwm}$
  note: $Ta_{pwm} = (T_{pwm}-T1_{pwm}-T2_{pwm})/2\\ Tb_{pwm} = Ta_{pwm}+T1_{pwm}\\ Tc_{pwm} = Tb_{pwm}+T2_{pwm}$
  note: $T1_{pwm}$
  note: $Tb_{pwm}$
  note: $Ta_{pwm}$
  note: $Tc_{pwm}$
  u_alpha_prime : Inport
  u_beta_prime : Inport  Port=2
  Tpwm : Inport  Port=3
  Action Port : ActionPort  ActionPortLabel=case [ 1 ]:
  Gain : Gain  Gain=1/sqrt(3)
  Gain1 : Gain  Gain=2/sqrt(3)
  Gain2 : Gain  Gain=1/2
  Mux : Mux  Inputs=3
  Product : Product
  Product1 : Product
  Sum : Sum  Inputs=|+-
  Sum1 : Sum  Inputs=--+
  Sum2 : Sum  Inputs=|++
  Sum3 : Sum  Inputs=++|
  tABC : Outport
  wires:
  u_beta_prime/1 -> Gain1/1, Gain/1
  u_alpha_prime/1 -> Sum/1
  Gain/1 -> Sum/2
  Sum/1 -> Product/1
  Tpwm/1 -> Sum1/3, Product1/2, Product/2
  Gain1/1 -> Product1/1
  Product/1 -> Sum1/1, Sum2/1
  Product1/1 -> Sum1/2, Sum3/2
  Sum1/1 -> Gain2/1
  Gain2/1 -> Mux/1, Sum2/2
  Sum2/1 -> Mux/2, Sum3/1
  Sum3/1 -> Mux/3
  Mux/1 -> tABC/1

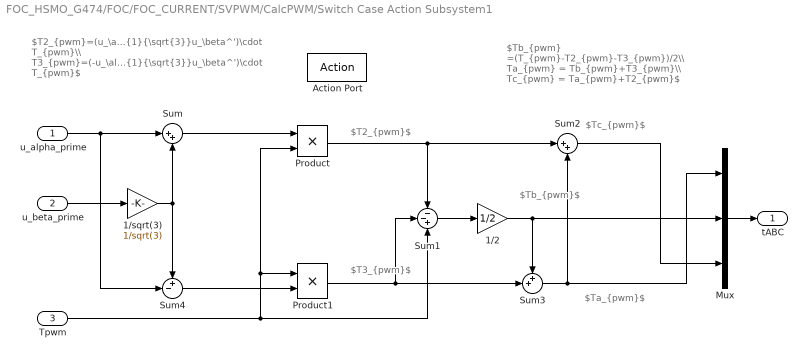
== system FOC_HSMO_G474/FOC/FOC_CURRENT/SVPWM/CalcPWM/Switch Case Action Subsystem1 ==
  note: $T2_{pwm}=(u_\alpha^'+\frac{1}{\sqrt{3}}u_\beta^')\cdot T_{pwm}\\ T3_{pwm}=(-u_\alpha^'+\frac{1}{\sqrt{3}}u_\beta^')\cdot T_{pwm}$
  note: $Tb_{pwm} =(T_{pwm}-T2_{pwm}-T3_{pwm})/2\\ Ta_{pwm} = Tb_{pwm}+T3_{pwm}\\ Tc_{pwm} = Ta_{pwm}+T2_{pwm}$
  note: $Ta_{pwm}$
  note: $Tc_{pwm}$
  note: $Tb_{pwm}$
  note: $T3_{pwm}$
  note: $T2_{pwm}$
  u_alpha_prime : Inport
  u_beta_prime : Inport  Port=2
  Tpwm : Inport  Port=3
  Action Port : ActionPort  ActionPortLabel=case [ 2 ]:
  1/2 : Gain  Gain=1/2
  1/sqrt(3) : Gain  Gain=1/sqrt(3)
  Mux : Mux  Inputs=3
  Product : Product  OutMin=0  OutMax=1e4
  Product1 : Product  OutMin=0  OutMax=1e4
  Sum : Sum  Inputs=|++  OutMin=0  OutMax=20
  Sum1 : Sum  Inputs=--+  OutMin=0  OutMax=2e4
  Sum2 : Sum  Inputs=|++  OutMin=0  OutMax=2e4
  Sum3 : Sum  Inputs=++|  OutMin=0  OutMax=2e4
  Sum4 : Sum  Inputs=+-|  OutMin=0  OutMax=20
  tABC : Outport
  wires:
  Sum/1 -> Product/1
  Sum4/1 -> Product1/2
  Tpwm/1 -> Sum1/3, Product/2, Product1/1
  1/2/1 -> Mux/2, Sum3/1
  Sum1/1 -> 1/2/1
  Sum2/1 -> Mux/3
  Sum3/1 -> Mux/1, Sum2/2
  u_beta_prime/1 -> 1/sqrt(3)/1
  1/sqrt(3)/1 -> Sum4/1, Sum/2
  u_alpha_prime/1 -> Sum4/2, Sum/1
  Mux/1 -> tABC/1
  Product/1 -> Sum1/1, Sum2/1
  Product1/1 -> Sum1/2, Sum3/2

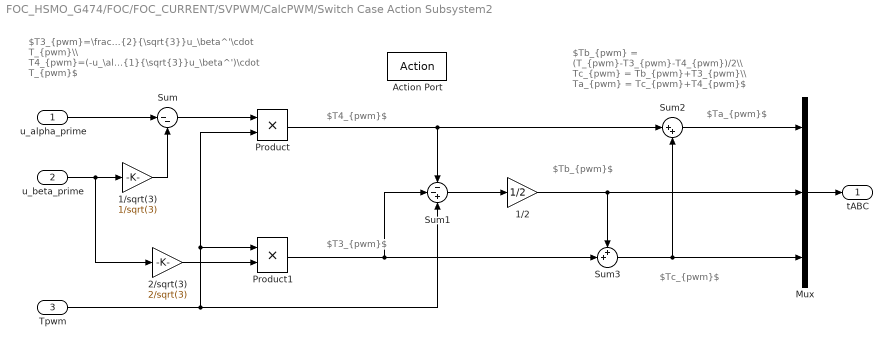
== system FOC_HSMO_G474/FOC/FOC_CURRENT/SVPWM/CalcPWM/Switch Case Action Subsystem2 ==
  note: $Tb_{pwm} = (T_{pwm}-T3_{pwm}-T4_{pwm})/2\\ Tc_{pwm} = Tb_{pwm}+T3_{pwm}\\ Ta_{pwm} = Tc_{pwm}+T4_{pwm}$
  note: $T3_{pwm}=\frac{2}{\sqrt{3}}u_\beta^'\cdot T_{pwm}\\ T4_{pwm}=(-u_\alpha^'-\frac{1}{\sqrt{3}}u_\beta^')\cdot T_{pwm}$
  note: $Tb_{pwm}$
  note: $Ta_{pwm}$
  note: $T3_{pwm}$
  note: $T4_{pwm}$
  note: $Tc_{pwm}$
  u_alpha_prime : Inport
  u_beta_prime : Inport  Port=2
  Tpwm : Inport  Port=3
  Action Port : ActionPort  ActionPortLabel=case [ 3 ]:
  1/2 : Gain  Gain=1/2
  1/sqrt(3) : Gain  Gain=1/sqrt(3)
  2/sqrt(3) : Gain  Gain=2/sqrt(3)
  Mux : Mux  Inputs=3
  Product : Product  OutMin=0  OutMax=1e4
  Product1 : Product  OutMin=0  OutMax=1e4
  Sum : Sum  Inputs=|--  OutMin=0  OutMax=20
  Sum1 : Sum  Inputs=--+  OutMin=0  OutMax=2e4
  Sum2 : Sum  Inputs=|++  OutMin=0  OutMax=2e4
  Sum3 : Sum  Inputs=++|  OutMin=0  OutMax=2e4
  tABC : Outport
  wires:
  Sum1/1 -> 1/2/1
  1/2/1 -> Sum3/1, Mux/2
  u_beta_prime/1 -> 2/sqrt(3)/1, 1/sqrt(3)/1
  2/sqrt(3)/1 -> Product1/2
  1/sqrt(3)/1 -> Sum/2
  u_alpha_prime/1 -> Sum/1
  Sum/1 -> Product/1
  Sum2/1 -> Mux/1
  Tpwm/1 -> Product/2, Product1/1, Sum1/3
  Sum3/1 -> Sum2/2, Mux/3
  Mux/1 -> tABC/1
  Product/1 -> Sum2/1, Sum1/1
  Product1/1 -> Sum3/2, Sum1/2

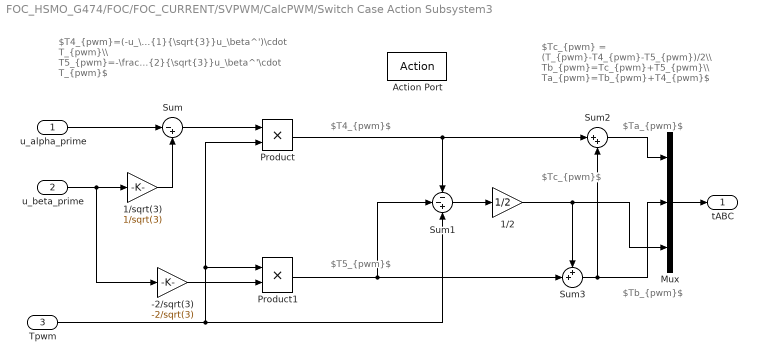
== system FOC_HSMO_G474/FOC/FOC_CURRENT/SVPWM/CalcPWM/Switch Case Action Subsystem3 ==
  note: $Tc_{pwm} = (T_{pwm}-T4_{pwm}-T5_{pwm})/2\\ Tb_{pwm}=Tc_{pwm}+T5_{pwm}\\ Ta_{pwm}=Tb_{pwm}+T4_{pwm}$
  note: $T4_{pwm}=(-u_\alpha^'+\frac{1}{\sqrt{3}}u_\beta^')\cdot T_{pwm}\\ T5_{pwm}=-\frac{2}{\sqrt{3}}u_\beta^'\cdot T_{pwm}$
  note: $Tc_{pwm}$
  note: $Ta_{pwm}$
  note: $T5_{pwm}$
  note: $T4_{pwm}$
  note: $Tb_{pwm}$
  u_alpha_prime : Inport
  u_beta_prime : Inport  Port=2
  Tpwm : Inport  Port=3
  Action Port : ActionPort  ActionPortLabel=case [ 4 ]:
  -2/sqrt(3) : Gain  Gain=-2/sqrt(3)
  1/2 : Gain  Gain=1/2
  1/sqrt(3) : Gain  Gain=1/sqrt(3)
  Mux : Mux  Inputs=3
  Product : Product  OutMin=0  OutMax=1e4
  Product1 : Product  OutMin=0  OutMax=1e4
  Sum : Sum  Inputs=|-+  OutMin=0  OutMax=20
  Sum1 : Sum  Inputs=--+  OutMin=0  OutMax=2e4
  Sum2 : Sum  Inputs=|++  OutMin=0  OutMax=2e4
  Sum3 : Sum  Inputs=++|  OutMin=0  OutMax=2e4
  tABC : Outport
  wires:
  Sum1/1 -> 1/2/1
  1/2/1 -> Sum3/1, Mux/3
  u_beta_prime/1 -> -2/sqrt(3)/1, 1/sqrt(3)/1
  1/sqrt(3)/1 -> Sum/2
  u_alpha_prime/1 -> Sum/1
  Sum/1 -> Product/1
  Sum2/1 -> Mux/1
  Tpwm/1 -> Sum1/3, Product/2, Product1/1
  Sum3/1 -> Sum2/2, Mux/2
  -2/sqrt(3)/1 -> Product1/2
  Mux/1 -> tABC/1
  Product1/1 -> Sum3/2, Sum1/2
  Product/1 -> Sum1/1, Sum2/1

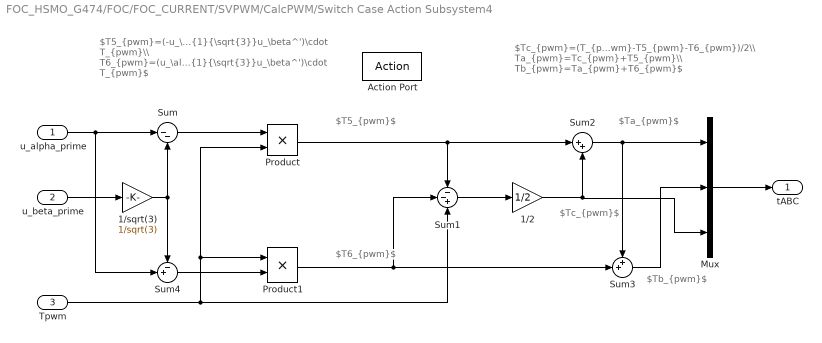
== system FOC_HSMO_G474/FOC/FOC_CURRENT/SVPWM/CalcPWM/Switch Case Action Subsystem4 ==
  note: $Tc_{pwm}=(T_{pwm}-T5_{pwm}-T6_{pwm})/2\\ Ta_{pwm}=Tc_{pwm}+T5_{pwm}\\ Tb_{pwm}=Ta_{pwm}+T6_{pwm}$
  note: $T5_{pwm}=(-u_\alpha^'-\frac{1}{\sqrt{3}}u_\beta^')\cdot T_{pwm}\\ T6_{pwm}=(u_\alpha^'-\frac{1}{\sqrt{3}}u_\beta^')\cdot T_{pwm}$
  note: $Tc_{pwm}$
  note: $Ta_{pwm}$
  note: $T6_{pwm}$
  note: $T5_{pwm}$
  note: $Tb_{pwm}$
  u_alpha_prime : Inport
  u_beta_prime : Inport  Port=2
  Tpwm : Inport  Port=3
  Action Port : ActionPort  ActionPortLabel=case [ 5 ]:
  1/2 : Gain  Gain=1/2
  1/sqrt(3) : Gain  Gain=1/sqrt(3)
  Mux : Mux  Inputs=3
  Product : Product  OutMin=0  OutMax=1e4
  Product1 : Product  OutMin=0  OutMax=1e4
  Sum : Sum  Inputs=|--  OutMin=0  OutMax=20
  Sum1 : Sum  Inputs=--+  OutMin=0  OutMax=2e4
  Sum2 : Sum  Inputs=|++  OutMin=0  OutMax=2e4
  Sum3 : Sum  Inputs=++|  OutMin=0  OutMax=2e4
  Sum4 : Sum  Inputs=-+|  OutMin=0  OutMax=20
  tABC : Outport
  wires:
  Sum1/1 -> 1/2/1
  1/2/1 -> Mux/3, Sum2/2
  u_beta_prime/1 -> 1/sqrt(3)/1
  Sum4/1 -> Product1/2
  1/sqrt(3)/1 -> Sum/2, Sum4/1
  u_alpha_prime/1 -> Sum4/2, Sum/1
  Sum/1 -> Product/1
  Sum2/1 -> Mux/1, Sum3/1
  Tpwm/1 -> Product/2, Product1/1, Sum1/3
  Sum3/1 -> Mux/2
  Mux/1 -> tABC/1
  Product1/1 -> Sum3/2, Sum1/2
  Product/1 -> Sum1/1, Sum2/1

== system FOC_HSMO_G474/FOC/FOC_CURRENT/SVPWM/CalcPWM/Switch Case Action Subsystem5 ==
  note: $Ta_{pwm}=(T_{pwm}-T6_{pwm}-T1_{pwm})/2\\ Tc_{pwm}=Ta_{pwm}+T1_{pwm}\\ Tb_{pwm}=Tc_{pwm}+T6_{pwm}$
  note: $T6_{pwm}=-\frac{2}{\sqrt{3}}u_\beta'\cdot T_{pwm}\\ T1_{pwm}=(u_\alpha^'+\frac{1}{\sqrt{3}}u_\beta')\cdot T_{pwm}$
  note: $Ta_{pwm}$
  note: $Tc_{pwm}$
  note: $T6_{pwm}$
  note: $T1_{pwm}$
  note: $Tb_{pwm}$
  u_alpha_prime : Inport
  u_beta_prime : Inport  Port=2
  Tpwm : Inport  Port=3
  Action Port : ActionPort  ActionPortLabel=case [ 6 ]:
  -2/sqrt(3) : Gain  Gain=-2/sqrt(3)
  1/2 : Gain  Gain=1/2
  1/sqrt(3) : Gain  Gain=1/sqrt(3)
  Mux : Mux  Inputs=3
  Product : Product  OutMin=0  OutMax=1e4
  Product1 : Product  OutMin=0  OutMax=1e4
  Sum : Sum  Inputs=|++  OutMin=0  OutMax=20
  Sum1 : Sum  Inputs=--+  OutMin=0  OutMax=2e4
  Sum2 : Sum  Inputs=|++  OutMin=0  OutMax=2e4
  Sum3 : Sum  Inputs=++|  OutMin=0  OutMax=2E4
  tABC : Outport
  wires:
  Sum1/1 -> 1/2/1
  1/2/1 -> Sum2/2, Mux/1
  u_beta_prime/1 -> -2/sqrt(3)/1, 1/sqrt(3)/1
  1/sqrt(3)/1 -> Sum/2
  u_alpha_prime/1 -> Sum/1
  Sum/1 -> Product/1
  Sum2/1 -> Sum3/1, Mux/3
  Sum3/1 -> Mux/2
  -2/sqrt(3)/1 -> Product1/2
  Mux/1 -> tABC/1
  Tpwm/1 -> Sum1/3, Product/2, Product1/1
  Product/1 -> Sum1/1, Sum2/1
  Product1/1 -> Sum3/2, Sum1/2

== system FOC_HSMO_G474/FOC/FOC_CURRENT/SVPWM/JudgeSector/If Action Subsystem ==
  note: $if(u_\alpha>0)\\ \quad if(\frac{1}{\sqrt{3}}u_\beta>u_\alpha)\\ \qquad sector=2\\ \quad else \\ \qquad sector=1\\ else \\ \quad if(-\frac{1}{\sqrt{3}}u_\beta>u_\alpha)\\ \qquad sector=3\\ \quad else\\ \qquad secotr = 2\\$
  u_alpha_prime : Inport
  u_beta_prime : Inport  Port=2
  Action Port : ActionPort  ActionPortLabel=if(u1)
  Constant : Constant  Value=0
  If : If  IfExpression=u1
  If Action Subsystem : Subsystem  TreatAsAtomicUnit=on
  If Action Subsystem1 : Subsystem  TreatAsAtomicUnit=on
  Merge : Merge
  Relational Operator : RelationalOperator  Operator=>  OutDataTypeStr=boolean  RndMeth=Simplest
  sector : Outport
  wires:
  u_alpha_prime/1 -> If Action Subsystem1/1(u_alpha_prime), If Action Subsystem/1(u_alpha_prime), Relational Operator/1
  Constant/1 -> Relational Operator/2
  Relational Operator/1 -> If/1
  If/1 -> If Action Subsystem/Action
  If/2 -> If Action Subsystem1/Action
  u_beta_prime/1 -> If Action Subsystem1/2(u_beta_prime), If Action Subsystem/2(u_beta_prime)
  If Action Subsystem/1(sector) -> Merge/1
  If Action Subsystem1/1(sector) -> Merge/2
  Merge/1 -> sector/1

== system FOC_HSMO_G474/FOC/FOC_CURRENT/SVPWM/JudgeSector/If Action Subsystem1 ==
  note: $if(u_\alpha>0)\\ \quad if(\frac{1}{\sqrt{3}}u_\beta>u_\alpha)\\ \quad sector = 5\\ \quad else\\ \qquad sector = 6\\ else \\ \quad if(\frac{1}{\sqrt{3}}u_\beta>u_\alpha)\\ \qquad sector = 4\\ \quad else\\ \qquad sector = 5$
  u_alpha_prime : Inport
  u_beta_prime : Inport  Port=2
  Action Port : ActionPort  ActionPortLabel=else
  Constant : Constant  Value=0
  If : If  IfExpression=u1
  If Action Subsystem : Subsystem  TreatAsAtomicUnit=on
  If Action Subsystem1 : Subsystem  TreatAsAtomicUnit=on
  Merge : Merge
  Relational Operator : RelationalOperator  Operator=>  OutDataTypeStr=boolean  RndMeth=Simplest
  sector : Outport
  wires:
  u_alpha_prime/1 -> If Action Subsystem1/1(u_alpha_prime), If Action Subsystem/1(u_alpha_prime), Relational Operator/1
  Constant/1 -> Relational Operator/2
  Relational Operator/1 -> If/1
  If/1 -> If Action Subsystem/Action
  If/2 -> If Action Subsystem1/Action
  u_beta_prime/1 -> If Action Subsystem/2(u_beta_prime), If Action Subsystem1/2(u_beta_prime)
  If Action Subsystem/1(sector) -> Merge/1
  If Action Subsystem1/1(sector) -> Merge/2
  Merge/1 -> sector/1
